simulink model "final_project_fixed_all"  (R2019b)
settings: Solver=FixedStepAuto  StartTime=0.0  StopTime=20  RelTol=1e-3  EnableMultiTasking=on
libraries: arduinolib x11, eePwmGenerator x2
settings Model: ExtModeTrigDuration=2  Creator=arash  LastModifiedBy=NavidN
settings SolverCC: AutoInsertRateTranBlk=on
settings OptimizationCC: EnhancedBackFolding=on  PassReuseOutputArgsAs=Individual arguments  ZeroExternalMemoryAtStartup=off  ZeroInternalMemoryAtStartup=off  MaxStackSize=64  OptimizeBlockOrder=speed  DifferentSizesBufferReuse=on  EfficientTunableParamExpr=on
settings DebuggingCC: ParameterTunabilityLossMsg=error  ArithmeticOperatorsInVariantConditions=warning
settings HardwareCC: ProdBitPerInt=16  ProdBitPerPointer=16  ProdBitPerSizeT=16  ProdBitPerPtrDiffT=16  ProdLargestAtomicFloat=None  ProdWordSize=8  ProdHWDeviceType=Atmel->AVR
settings SFSimCC: MATLABDynamicMemAlloc=off  CustomCodeUndefinedFunction=UseInterfaceOnly
settings RTWCC: SystemTargetFile=ert.tlc  HardwareBoard=Arduino Uno  TLCOptions=-aInlineSetEventsForThisBaseRateFcn=TLC_FALSE -aSuppressMultiTaskScheduler=TLC_FALSE -aRateBasedStepFcn=1  PackageName=final  TemplateMakefile=ert_default_tmf  GenerateReport=on  Toolchain=Arduino AVR  BuildConfiguration=Faster Runs  IncludeHyperlinkInReport=on  LaunchReport=on  GenerateTraceInfo=on  GenerateTraceReport=on  GenerateTraceReportSl=on  GenerateTraceReportSf=on  GenerateTraceReportEml=on
settings CodeAppCC: ForceParamTrailComments=on  IgnoreCustomStorageClasses=off  OperatorAnnotations=on  SimulinkDataObjDesc=on  SFDataObjDesc=on  InsertBlockDesc=on
settings ERTTargetCC: SupportContinuousTime=on  SupportVariableSizeSignals=on  ExtModeStaticAllocSize=250

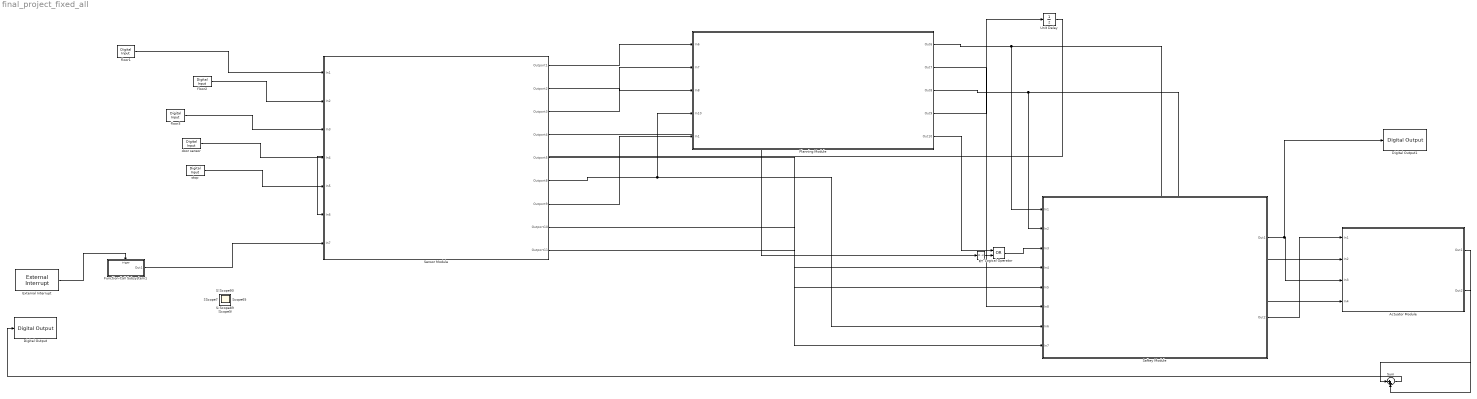
== system final_project_fixed_all ==
  "Actuator Module " : Subsystem
  Digital Output : arduinolib/Digital Output  pinNumber=9  blockPlatform=arduino
  Digital Output1 : arduinolib/Digital Output  pinNumber=7  blockPlatform=arduino
  External Interrupt : arduinolib/External Interrupt  Pin=2  PullUp=off  Mode=RISING  InterruptSimulationInput=off
      settings: SourceProductName=Simulink Support Package for Arduino Hardware  SourceProductBaseCode=ARDUINO
  Function-Call Subsystem1 : Subsystem  TreatAsAtomicUnit=on
  Logical Operator : Logic  Operator=OR  AllPortsSameDT=off  OutDataTypeStr=boolean
  Planning Module : Subsystem
  RT : RateTransition
  Saftey Module : Subsystem
  "Sensor Module " : Subsystem
  Sum : Sum  Inputs=|++
  Unit Delay : UnitDelay  SampleTime=-1  HasFrameUpgradeWarning=on
  door sensor : arduinolib/Digital Input  pinNumber=8  SampleTime=0.001  blockPlatform=arduino
      settings: SourceProductName=Simulink Support Package for Arduino Hardware
  floor1 : arduinolib/Digital Input  pinNumber=4  SampleTime=0.001  blockPlatform=arduino
      settings: SourceProductName=Simulink Support Package for Arduino Hardware
  floor2 : arduinolib/Digital Input  pinNumber=5  SampleTime=0.001  blockPlatform=arduino
      settings: SourceProductName=Simulink Support Package for Arduino Hardware
  floor3 : arduinolib/Digital Input  pinNumber=6  SampleTime=0.001  blockPlatform=arduino
      settings: SourceProductName=Simulink Support Package for Arduino Hardware
  stop : arduinolib/Digital Input  pinNumber=3  SampleTime=0.001  blockPlatform=arduino
      settings: SourceProductName=Simulink Support Package for Arduino Hardware
  Scope{,1..26} (27 alike) : Scope
  wires:
  "Sensor Module "/6(Outport8) -> Saftey Module/7(In6), Planning Module/4(In10)
  "Sensor Module "/8(Outport10) -> Saftey Module/4(In4)
  Logical Operator/1 -> Saftey Module/3(In3)
  "Sensor Module "/4(Outport4) -> RT/1
  "Sensor Module "/5(Outport5) -> Saftey Module/5(In5)
  "Sensor Module "/9(Outport11) -> Saftey Module/8(In7)
  Planning Module/1(Out6) -> "Actuator Module "/2(In2), Saftey Module/1(In1)
  Planning Module/2(Out7) -> Saftey Module/6(In8)
  Planning Module/3(Out8) -> "Actuator Module "/4(In4), Saftey Module/2(In2)
  Planning Module/5(Out10) -> Logical Operator/1
  Planning Module/4(Out9) -> Unit Delay/1
  "Sensor Module "/1(Outport1) -> Planning Module/1(In6)
  "Sensor Module "/2(Outport2) -> Planning Module/3(In8)
  "Sensor Module "/3(Outport3) -> Planning Module/2(In7)
  "Sensor Module "/7(Outport9) -> Planning Module/5(In1)
  "Actuator Module "/1(Out1) -> Sum/1
  "Actuator Module "/2(Out2) -> Sum/2
  Unit Delay/1 -> "Sensor Module "/6(In6)
  floor1/1 -> "Sensor Module "/1(In1)
  door sensor/1 -> "Sensor Module "/4(In4)
  stop/1 -> "Sensor Module "/5(In5)
  floor3/1 -> "Sensor Module "/3(In3)
  floor2/1 -> "Sensor Module "/2(In2)
  Sum/1 -> Digital Output/1
  Function-Call Subsystem1/1(Out1) -> "Sensor Module "/7(In7)
  External Interrupt/1 -> Function-Call Subsystem1/Trigger
  Saftey Module/2(Out2) -> "Actuator Module "/1(In1)
  Saftey Module/1(Out1) -> Digital Output1/1, "Actuator Module "/3(In3)
  RT/1 -> Logical Operator/2

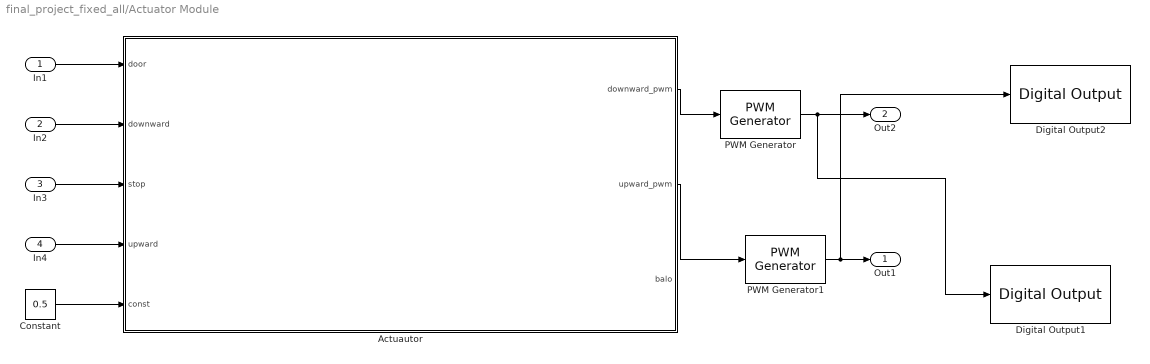
== system final_project_fixed_all/Actuator Module  ==
  In1 : Inport
  In2 : Inport  Port=2
  In3 : Inport  Port=3
  In4 : Inport  Port=4
  "Actuautor " : Stateflow chart  TreatAsAtomicUnit=on
  Constant : Constant  Value=0.5
  Digital Output1 : arduinolib/Digital Output  pinNumber=11  blockPlatform=arduino
  Digital Output2 : arduinolib/Digital Output  pinNumber=10  blockPlatform=arduino
  PWM Generator : eePwmGenerator/PWM Generator  CarrCount=Up  Tper=0.02  Ts=5e-5
      settings: SourceProductName=Simscape Electrical
  PWM Generator1 : eePwmGenerator/PWM Generator  CarrCount=Up  Tper=0.02  Ts=5e-5
      settings: SourceProductName=Simscape Electrical
  Out1 : Outport  VectorParamsAs1DForOutWhenUnconnected=off
  Out2 : Outport  Port=2  VectorParamsAs1DForOutWhenUnconnected=off
  wires:
  In1/1 -> "Actuautor "/1(door)
  In2/1 -> "Actuautor "/2(downward)
  In3/1 -> "Actuautor "/3(stop)
  In4/1 -> "Actuautor "/4(upward)
  Constant/1 -> "Actuautor "/5(const)
  PWM Generator/1 -> Digital Output1/1, Out2/1
  "Actuautor "/1(downward_pwm) -> PWM Generator/1
  "Actuautor "/2(upward_pwm) -> PWM Generator1/1
  PWM Generator1/1 -> Digital Output2/1, Out1/1

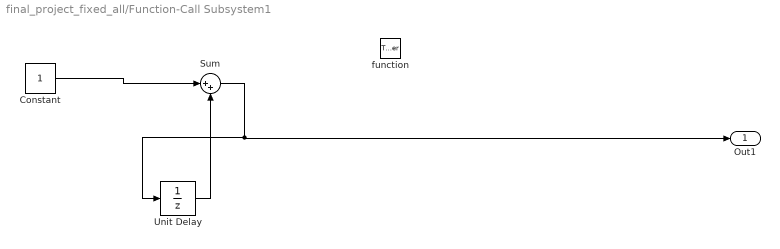
== system final_project_fixed_all/Function-Call Subsystem1 ==
  function : TriggerPort  TriggerType=function-call  VariantControl=Variant
  Constant : Constant
  Sum : Sum  Inputs=|++
  Unit Delay : UnitDelay  SampleTime=-1  HasFrameUpgradeWarning=on
  Out1 : Outport  VectorParamsAs1DForOutWhenUnconnected=off
  wires:
  Constant/1 -> Sum/1
  Sum/1 -> Out1/1, Unit Delay/1
  Unit Delay/1 -> Sum/2

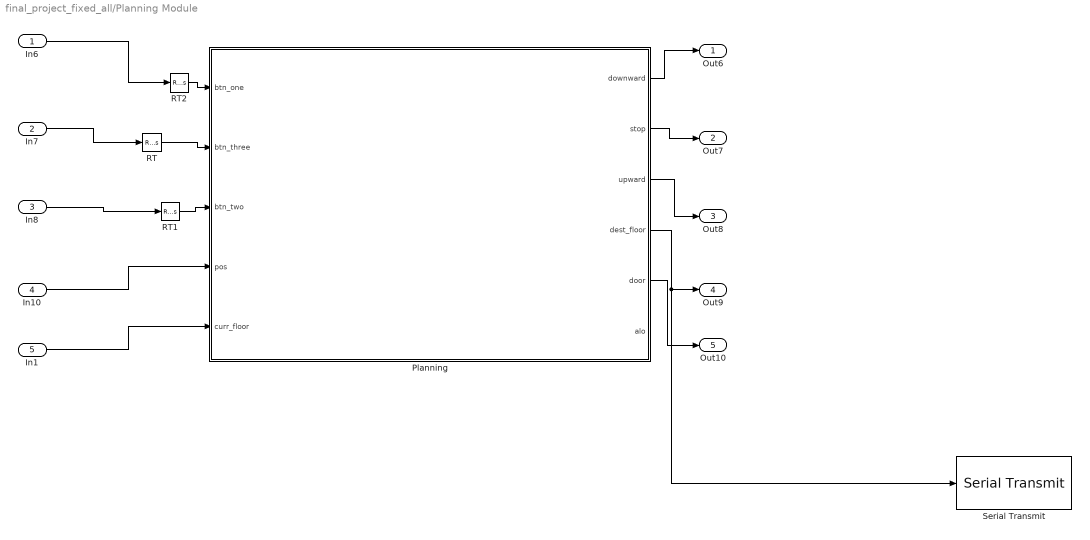
== system final_project_fixed_all/Planning Module ==
  In6 : Inport
  In7 : Inport  Port=2
  In8 : Inport  Port=3
  In10 : Inport  Port=4
  In1 : Inport  Port=5
  "Planning " : Stateflow chart  TreatAsAtomicUnit=on
  RT : RateTransition
  RT1 : RateTransition  OutPortSampleTime=5e-05
  RT2 : RateTransition  OutPortSampleTime=5e-05
  Serial Transmit : arduinolib/Serial Transmit  portNumber=0  sendmode=println  label=dst :  sendformat=Decimal  floatprecision=2  blockPlatform=arduino
      settings: SourceProductName=Simulink Support Package for Arduino Hardware
  Out6 : Outport  VectorParamsAs1DForOutWhenUnconnected=off
  Out7 : Outport  Port=2  VectorParamsAs1DForOutWhenUnconnected=off
  Out8 : Outport  Port=3  VectorParamsAs1DForOutWhenUnconnected=off
  Out9 : Outport  Port=4  VectorParamsAs1DForOutWhenUnconnected=off
  Out10 : Outport  Port=5  VectorParamsAs1DForOutWhenUnconnected=off
  wires:
  "Planning "/3(upward) -> Out8/1
  In8/1 -> RT1/1
  In6/1 -> RT2/1
  "Planning "/4(dest_floor) -> Serial Transmit/1, Out9/1
  In10/1 -> "Planning "/4(pos)
  "Planning "/1(downward) -> Out6/1
  In7/1 -> RT/1
  "Planning "/5(door) -> Out10/1
  "Planning "/2(stop) -> Out7/1
  In1/1 -> "Planning "/5(curr_floor)
  RT/1 -> "Planning "/2(btn_three)
  RT1/1 -> "Planning "/3(btn_two)
  RT2/1 -> "Planning "/1(btn_one)

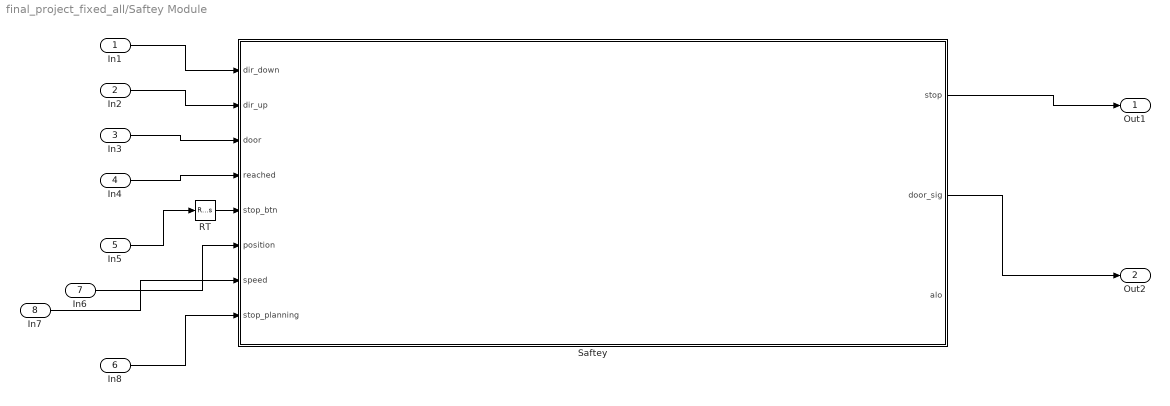
== system final_project_fixed_all/Saftey Module ==
  In1 : Inport
  In2 : Inport  Port=2
  In3 : Inport  Port=3
  In4 : Inport  Port=4
  In5 : Inport  Port=5
  In8 : Inport  Port=6
  In6 : Inport  Port=7
  In7 : Inport  Port=8
  RT : RateTransition
  "Saftey " : Stateflow chart  TreatAsAtomicUnit=on
  Out1 : Outport  VectorParamsAs1DForOutWhenUnconnected=off
  Out2 : Outport  Port=2  VectorParamsAs1DForOutWhenUnconnected=off
  wires:
  In2/1 -> "Saftey "/2(dir_up)
  In3/1 -> "Saftey "/3(door)
  In4/1 -> "Saftey "/4(reached)
  In5/1 -> RT/1
  In1/1 -> "Saftey "/1(dir_down)
  "Saftey "/1(stop) -> Out1/1
  In6/1 -> "Saftey "/6(position)
  In7/1 -> "Saftey "/7(speed)
  "Saftey "/2(door_sig) -> Out2/1
  In8/1 -> "Saftey "/8(stop_planning)
  RT/1 -> "Saftey "/5(stop_btn)

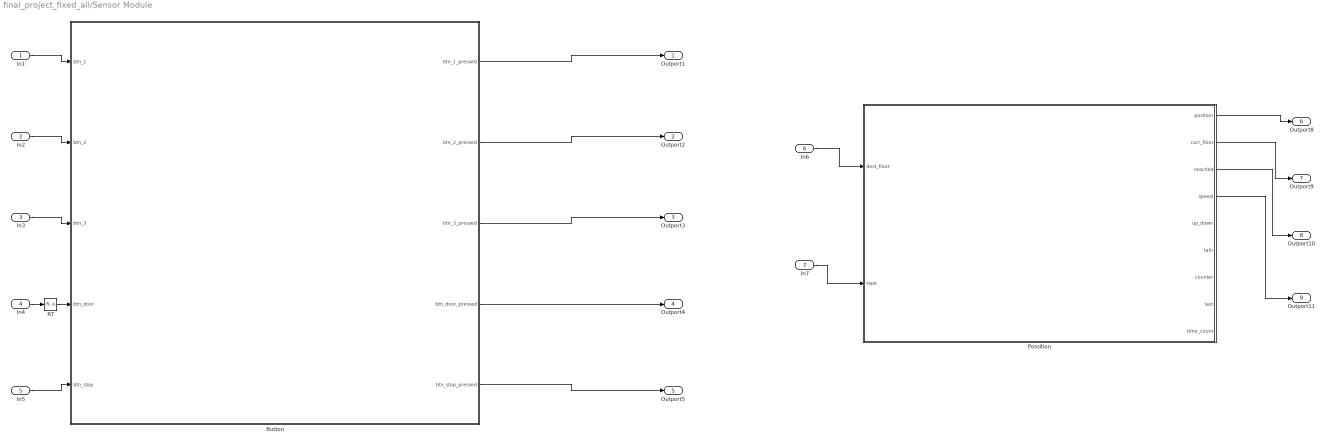
== system final_project_fixed_all/Sensor Module  ==
  In1 : Inport
  In2 : Inport  Port=2
  In3 : Inport  Port=3
  In4 : Inport  Port=4
  In5 : Inport  Port=5
  In6 : Inport  Port=6
  In7 : Inport  Port=7
  "Button " : Stateflow chart  TreatAsAtomicUnit=on
  Possition : Stateflow chart  TreatAsAtomicUnit=on
  RT : RateTransition  OutPortSampleTime=0.001
  Outport1 : Outport
  Outport2 : Outport  Port=2
  Outport3 : Outport  Port=3
  Outport4 : Outport  Port=4
  Outport5 : Outport  Port=5
  Outport8 : Outport  Port=6
  Outport9 : Outport  Port=7
  Outport10 : Outport  Port=8
  Outport11 : Outport  Port=9
  wires:
  "Button "/1(btn_1_pressed) -> Outport1/1
  "Button "/2(btn_2_pressed) -> Outport2/1
  "Button "/5(btn_stop_pressed) -> Outport5/1
  "Button "/4(btn_door_pressed) -> Outport4/1
  "Button "/3(btn_3_pressed) -> Outport3/1
  Possition/1(position) -> Outport8/1
  Possition/3(reached) -> Outport10/1
  Possition/4(speed) -> Outport11/1
  In1/1 -> "Button "/1(btn_1)
  In2/1 -> "Button "/2(btn_2)
  In3/1 -> "Button "/3(btn_3)
  In4/1 -> RT/1
  In5/1 -> "Button "/5(btn_stop)
  In6/1 -> Possition/1(dest_floor)
  In7/1 -> Possition/2(tape)
  Possition/2(curr_floor) -> Outport9/1
  RT/1 -> "Button "/4(btn_door)

== stateflow chart final_project_fixed_all/Sensor Module /Possition ==
  state NOT_INIT
    state POSITION_CALCULATION [parallel]
      settings: executionOrder=1
      (history)
      state NOT_MOVING
        entry :
        counter = 0;
        up_down = 0;
        position = (curr_floor - 1) * 400;
        last_pos = position;
        reached = 1;
        speed = 0;
        talo = 0;
      state NOT_EQUAL
        entry :
        last = (tape);
      state MOVING
        entry :
        position = ((curr_floor - 1) * 400) + up_down * counter;
        dir_up = max(up_down, 0);
        dir_down = max(-up_down ,0);
        reached = 0;
      state ONE_FLOOR_REACHED
        entry:
        counter = 0;
        curr_floor = curr_floor + up_down;
        talo = tape + last;
      state NOT_EQUAL2
        entry:
        last = (tape);
        counter = counter + 1;
      NOT_MOVING -> MOVING [order 1] : [curr_floor > dest_floor && dest_floor ~= -1]{up_down = -1}
      (default) -> NOT_MOVING
      NOT_MOVING -> MOVING [order 2] : [curr_floor < dest_floor && dest_floor ~= -1]{up_down = 1}
      MOVING -> NOT_MOVING [order 1] : [dest_floor == -1]
      MOVING -> NOT_EQUAL [order 2] : [(tape) ~= last]
      ONE_FLOOR_REACHED -> MOVING
      NOT_EQUAL -> NOT_EQUAL [order 2] : [(tape) == last]
      NOT_EQUAL2 -> MOVING [order 2] : [counter < 400]
      NOT_EQUAL -> NOT_EQUAL2 [order 1] : [ (tape) ~= last]
      NOT_EQUAL2 -> ONE_FLOOR_REACHED [order 1] : [counter >= 400]
    state SPEED_CALC [parallel]
      settings: executionOrder=2
      (history)
      state Speed
        entry:
        speed = abs(position-last_pos);
        last_pos = position;
      (default) -> Speed
      Speed -> Speed : after(1,sec)
  state SPEED [commented out]
    entry:
  state INIT
    entry:
    curr_floor = 1;
    last_pos = 0;
    last = 0;
    talo = 0;
    time_count = 0;
  state Speed2 [commented out]
    entry:
    speed =( abs(position - last_pos)*  500)/ time_count;
    last_pos = position;
  (default) -> SPEED [commented out]
  (default) -> INIT
  INIT -> NOT_INIT
  Speed2 -> SPEED [commented out] : {time_count = 0;}
  SPEED -> Speed2 [commented out] : [after(10, msec) && ( position ~= last_pos || time_count > 10)]
  SPEED -> SPEED [commented out] : [after(2, msec) && (position == last_pos ) && time_count <=10 ]{time_count = time_count + 1 ;}
  data: dest_floor input; tape input; position output; curr_floor output; reached output; last_pos local; speed output; dir_down local; dir_up local; up_down output; talo output; counter output; last output; time_count output

== stateflow chart final_project_fixed_all/Saftey Module/Saftey  ==
  state POSITION_DOWN
    entry :
    stop = 1;
    alo = 5;
  state MONITOR
    during:
    stop = 0;
    alo = 0;
  state POSITION_TOP
    entry :
    stop = 1;
    alo = 4;
  state DOOR
    entry :
    stop = 1;
    door_sig = 1;
    alo = 1;
  state STOP_BTN
    entry :
    stop = 1;
    alo = 2;
  state SPEED
    entry :
    stop = 1;
    alo = 3;
  MONITOR -> POSITION_DOWN [order 5] : [after (0.1, msec) && position == 0 && reached == 0 && dir_down == 1]
  (default) -> MONITOR
  POSITION_DOWN -> MONITOR [order 2] : [after (0.1, msec)  &&( reached == 1 || dir_down == 0)]
  MONITOR -> POSITION_TOP [order 3] : [after (0.1, msec) && position == 10 && reached == 0 && dir_up == 1]
  MONITOR -> DOOR [order 1] : [after(0.1, msec) && door == 1 && reached ==0]
  DOOR -> MONITOR [order 2] : [after(0.1, msec) && door == 0]{door_sig = 0;}
  POSITION_TOP -> MONITOR [order 1] : [after (0.1, msec)  &&( reached == 1 || dir_up == 0)]
  MONITOR -> SPEED [order 4] : [after (0.1, msec) && speed > 5000]
  MONITOR -> STOP_BTN [order 2] : [( stop_btn == 1 || stop_planning == 1) ]
  STOP_BTN -> MONITOR [order 2] : [after (0.1, msec) &&(stop_planning == 0)]
  SPEED -> MONITOR [order 1] : [after (0.1, msec) && speed <= 5000]
  POSITION_DOWN -> POSITION_DOWN [order 1] : [after (10, msec) && position == 10 && reached == 0 && dir_up == 1]
  POSITION_TOP -> POSITION_TOP [order 2] : [after (0.1, msec) && position == 10 && reached == 0 && dir_up == 1]
  DOOR -> DOOR [order 1] : [after(0.1, msec) && door == 1]
  SPEED -> SPEED [order 2] : [after (0.1, msec) && speed > 5000]
  STOP_BTN -> STOP_BTN [order 1] : [after(3, msec) && (stop_btn == 1 || stop_planning == 0)]
  data: dir_down input; dir_up input; door input; reached input; stop_btn input; stop output; position input; speed input; door_sig output; stop_planning input; alo output

== stateflow chart final_project_fixed_all/Sensor Module /Button  ==
  state TIMER_DOOR
  state BTN_DOOR_PRESSED
    entry:
    btn_door_pressed = 1;
  state TIMER_1
  state IDLE
    entry:
    btn_1_pressed = 0;
    btn_2_pressed = 0;
    btn_3_pressed = 0;
    btn_stop_pressed = 0;
    btn_door_pressed = 0;
  state BTN_1_PRESSED
    entry:
    btn_1_pressed = 1;
  state TIMER_STOP
  state TIMER_2
  state TIMER_3
  state BTN_STOP_PRESSED
    entry:
    btn_stop_pressed = 1;
  state BTN_2_PRESSED
    entry:
    btn_2_pressed = 1;
  state BTN_3_PRESSED3
    entry:
    btn_3_pressed = 1;
  TIMER_DOOR -> BTN_DOOR_PRESSED [order 1] : [btn_door == 1 && after (2, msec)]
  TIMER_DOOR -> IDLE [order 2] : [btn_door == 0]
  IDLE -> TIMER_1 [order 1] : [btn_1 == 1]
  IDLE -> TIMER_DOOR [order 5] : [btn_door == 1]
  BTN_DOOR_PRESSED -> IDLE : [after(0.1,msec)]
  TIMER_1 -> IDLE [order 2] : [btn_1 == 0]
  (default) -> IDLE
  TIMER_1 -> BTN_1_PRESSED [order 1] : [btn_1 == 1 && after(2, msec)]
  BTN_STOP_PRESSED -> IDLE : [after(10,sec)]
  IDLE -> TIMER_STOP [order 4] : [btn_stop == 1]
  TIMER_STOP -> IDLE [order 2] : [btn_stop == 0]
  BTN_1_PRESSED -> IDLE
  BTN_2_PRESSED -> IDLE
  IDLE -> TIMER_2 [order 2] : [btn_2 == 1]
  TIMER_2 -> IDLE [order 2] : [btn_2== 0]
  IDLE -> TIMER_3 [order 3] : [btn_3 == 1]
  TIMER_3 -> IDLE [order 2] : [btn_3== 0]
  BTN_3_PRESSED3 -> IDLE
  TIMER_STOP -> BTN_STOP_PRESSED [order 1] : [btn_stop == 1 && after (2, msec)]
  TIMER_2 -> BTN_2_PRESSED [order 1] : [btn_2 == 1 && after (2, msec)]
  TIMER_3 -> BTN_3_PRESSED3 [order 1] : [btn_3 == 1 && after (2, msec)]
  data: btn_1 input; btn_2 input; btn_3 input; btn_door input; btn_stop input; btn_1_pressed output; btn_2_pressed output; btn_3_pressed output; btn_door_pressed output; btn_stop_pressed output

== stateflow chart final_project_fixed_all/Actuator Module /Actuautor  ==
  state NOT_STOP
    entry:
    balo = 0;
  state STOP
    entry:
    balo = 1
    upward_pwm = 0;
    downward_pwm = 0;
  STOP -> NOT_STOP [order 2] : [stop == 0 && door == 0 && downward ==1 ]{downward_pwm = const}
  NOT_STOP -> STOP : [stop == 1 || door == 1]
  STOP -> NOT_STOP [order 1] : [stop == 0 && door == 0 && upward ==1 ]{upward_pwm = const}
  (default) -> STOP
  data: door input; downward input; stop input; upward input; downward_pwm output; upward_pwm output; const input double; balo output

== stateflow chart final_project_fixed_all/Planning Module/Planning  ==
  state NOT_INIT
    state INPUT [parallel]
      settings: executionOrder=1
      state btn_read
      (default) -> btn_read
      btn_read -> btn_read [order 3] : [ btn_three == 1]{three_pressed = 1;}
      btn_read -> btn_read [order 2] : [ btn_two == 1]{two_pressed = 1;}
      btn_read -> btn_read [order 1] : [ btn_one == 1]{one_pressed = 1;}
    state PLANNING [parallel]
      settings: executionOrder=3
      state IDLE
      state MOVE_DOWN
        entry:
        upward =0;
        downward = 1;
      state MOVE_UP
        entry:
        downward = 0;
        upward = 1;
      (default) -> IDLE
      IDLE -> MOVE_UP [order 2] : [dest_floor > curr_floor]
      IDLE -> MOVE_DOWN [order 1] : [dest_floor ~= -1 && dest_floor < curr_floor]
      MOVE_DOWN -> IDLE [order 2] : [curr_floor == dest_floor && dest_floor == 1]{downward=0;dest_floor = -1;one_pressed = 0;}
      MOVE_UP -> IDLE [order 3] : [curr_floor == dest_floor && dest_floor == 1]{upward=0;dest_floor = -1;one_pressed = 0;}
      MOVE_DOWN -> IDLE [order 3] : [curr_floor == dest_floor && dest_floor == 3]{downward=0;dest_floor = -1;three_pressed = 0;}
      MOVE_DOWN -> IDLE [order 1] : [curr_floor == dest_floor && dest_floor == 2]{downward=0;dest_floor = -1;two_pressed = 0;}
      MOVE_UP -> IDLE [order 2] : [curr_floor == dest_floor && dest_floor == 3]{upward=0;dest_floor = -1;three_pressed = 0;}
      MOVE_UP -> IDLE [order 1] : [curr_floor == dest_floor && dest_floor == 2]{upward=0;dest_floor = -1;two_pressed = 0;}
    state DESTINATION [parallel]
      settings: executionOrder=2
      state NOT_MOVING
        entry:
        alo = 1
        stop = 0;
        door = 0;
      state F2
        entry:
        dest_floor = 2
      state F3
        entry:
        dest_floor = 3
      state F1
        entry:
        dest_floor = 1
      state MOVING
      state REACH_FLOOR
        entry:
        door = 1;
        stop = 1;
      REACH_FLOOR -> NOT_MOVING : [after(1,msec)]{door = 0; stop = 0;}
      (default) -> NOT_MOVING
      NOT_MOVING -> F2 [order 4] : [curr_floor == 3 && two_pressed == 1 ]
      NOT_MOVING -> F1 [order 6] : [curr_floor == 3 && one_pressed == 1 && two_pressed == 0]
      NOT_MOVING -> F2 [order 1] : [curr_floor == 1 && two_pressed == 1 ]{alo = 0}
      NOT_MOVING -> F1 [order 3] : [curr_floor == 2 && one_pressed == 1 && three_pressed == 0 ]
      NOT_MOVING -> F3 [order 5] : [curr_floor == 2 && three_pressed ==  1]{alo = 0}
      NOT_MOVING -> F3 [order 2] : [curr_floor == 1 && two_pressed == 0 && three_pressed ==  1]
      F2 -> MOVING
      F3 -> MOVING
      F1 -> MOVING
      MOVING -> MOVING [order 2] : [two_pressed == 1 && dest_floor == 3 && pos < 200]{dest_floor = 2}
      MOVING -> REACH_FLOOR [order 3] : [dest_floor == -1]
      MOVING -> MOVING [order 1] : [two_pressed == 1 && dest_floor == 1 && pos > 600]{dest_floor = 2}
  state INIT
    entry:
    one_pressed = 0;
    two_pressed = 0;
    three_pressed = 0;
    dest_floor = -1;
    alo = 0;
  (default) -> INIT
  INIT -> NOT_INIT
  data: btn_one input; btn_three input; btn_two input; one_pressed local; three_pressed local; two_pressed local; downward output; stop output; upward output; dest_floor output; door output; pos input; curr_floor input; alo output
